simulink model "sfcndemo_port_triggered"  (Simulink 7.6)
settings: Solver=FixedStepDiscrete  SolverMode=SingleTasking  StartTime=0.0  StopTime=10.0  RelTol=1e-3
Description:
  | Port-Based Sample Time C-MEX S-function, suitable for use standalone or inside any type of triggered subsystem
settings Model: Creator=The MathWorks Inc.  ExtModeAutoUpdateStatusClock=off
settings OptimizationCC: BooleanDataType=off  InitFltsAndDblsToZero=on
settings DebuggingCC: SaveWithParameterizedLinksMsg=none  SignalResolutionControl=TryResolveAllWithWarning  SolverPrmCheckMsg=none  MultiTaskDSMMsg=warning  MultiTaskCondExecSysMsg=none
settings HardwareCC: TargetUnknown=on
settings RTWCC: IncludeERTFirstTime=on
settings CodeAppCC: CustomSymbolStrFcn=$F$N$M
settings GRTTargetCC: TargetFcnLib=ansi_tfl_tmw.mat

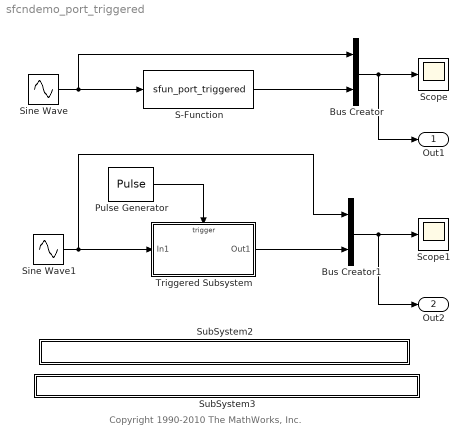
== system sfcndemo_port_triggered ==
  note: Copyright 1990-2010 The MathWorks, Inc.
  Bus Creator : BusCreator  Inputs=2
  Bus Creator1 : BusCreator  Inputs=2
  Pulse Generator : DiscretePulseGenerator  PulseType=Time based  PulseWidth=50
  S-Function : S-Function  FunctionName=sfun_port_triggered  Parameters=10  EnableBusSupport=off
  Scope : Scope
      settings: TimeRange=10  YMin=-1  YMax=1
  Scope1 : Scope
      settings: TimeRange=10  YMin=-1  YMax=1
  Sine Wave : Sin  SampleTime=0.1
  Sine Wave1 : Sin  SampleTime=0
  SubSystem2 : Subsystem  mask{filename=sfun_port_triggered.c}
      mask init:
      | x=sfundemo_maskdisp;
      settings: AttributesFormatString=\n  OpenFcn=sfundemo_openfcn
      mask Display: disp(x);
  SubSystem3 : Subsystem  mask{filename=sfun_port_triggered.tlc}
      mask init:
      | x=sfundemo_maskdisp;
      settings: AttributesFormatString=\n  OpenFcn=sfundemo_openfcn
      mask Display: disp(x);
  Triggered Subsystem : Subsystem  TreatAsAtomicUnit=on
  Out1 : Outport
  Out2 : Outport  Port=2
  wires:
  Pulse Generator/1 -> Triggered Subsystem/Trigger
  Sine Wave/1 -> S-Function/1, Bus Creator/1
  S-Function/1 -> Bus Creator/2
  Bus Creator/1 -> Scope/1, Out1/1
  Bus Creator1/1 -> Scope1/1, Out2/1
  Sine Wave1/1 -> Triggered Subsystem/1(In1), Bus Creator1/1
  Triggered Subsystem/1(Out1) -> Bus Creator1/2

== system sfcndemo_port_triggered/SubSystem2 ==

== system sfcndemo_port_triggered/SubSystem3 ==

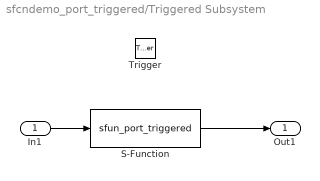
== system sfcndemo_port_triggered/Triggered Subsystem ==
  In1 : Inport
  Trigger : TriggerPort
  S-Function : S-Function  FunctionName=sfun_port_triggered  Parameters=2  EnableBusSupport=off
  Out1 : Outport
  wires:
  In1/1 -> S-Function/1
  S-Function/1 -> Out1/1
